simulink model "PSK8"  (R2017a)
settings: Solver=VariableStepAuto  StartTime=0.0  StopTime=9600*Tb  RelTol=1e-3
values from neighbouring files (symbols this model uses):
  Tb = 5e-8    (= 5e-08)    [cuatrobits.m]    (also in dosbits.m; seisbits.m; tresbits.m)
libraries: commfilt2 x4, commdigbbndpm3 x2, dspsigops x2, simulink x1
settings Model: Creator=se.alfonso  LastModifiedBy=af.diaz16

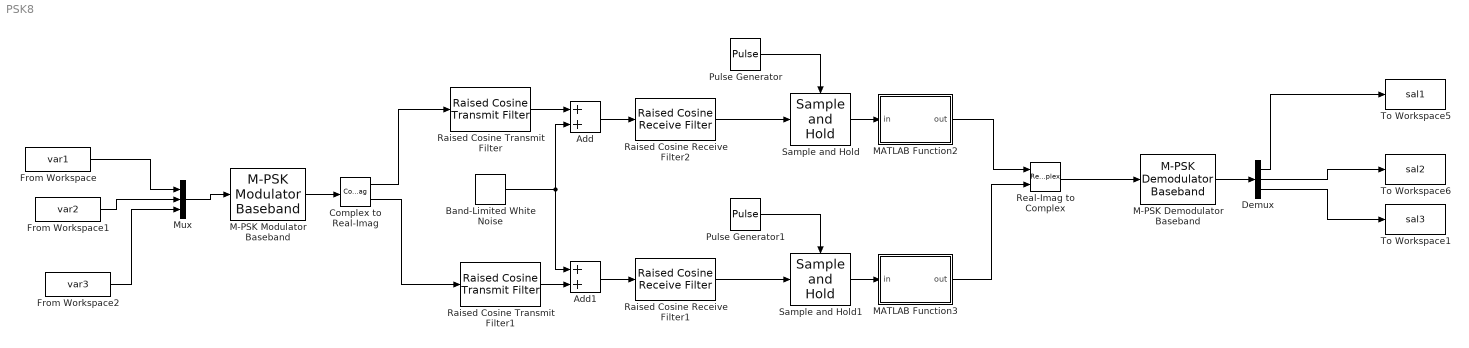
== system PSK8 ==
  Add : Sum
  Add1 : Sum
  Band-Limited White Noise : simulink/Sources/Band-Limited White Noise  Cov=No  Ts=Tb  seed=[23341]
  Complex to Real-Imag : ComplexToRealImag
  Demux : Demux  Outputs=3
  From Workspace : FromWorkspace  VariableName=var1  SampleTime=Tb
  From Workspace1 : FromWorkspace  VariableName=var2  SampleTime=Tb
  From Workspace2 : FromWorkspace  VariableName=var3  SampleTime=Tb
  M-PSK Demodulator Baseband : commdigbbndpm3/M-PSK Demodulator Baseband  M=8  OutType=Bit  DecType=Hard decision  VarSource=Dialog  Variance=1  Dec=Gray  Mapping=[0:7]  Ph=pi/8  outDtype1=Inherit via internal rule  outDtype2=Inherit via internal rule  derotateFactorWordLen=16  derotateFactorDataTypeStr=Inherit: Same word length as input  derotateFactorLastDataTypeStr=Inherit: Same word length as input
      settings: SourceProductName=Communications System Toolbox
  M-PSK Modulator Baseband : commdigbbndpm3/M-PSK Modulator Baseband  M=8  InType=Bit  Enc=Gray  Mapping=[0:7]  Ph=pi/8  outDtype=double  outWordLen=16  outUDDataType=sfix(16)  outFracLenMode=Best precision  outFracLen=15  outDataTypeStr=double  outLastDataTypeStr=double
      settings: SourceProductName=Communications System Toolbox
  MATLAB Function2 : MATLAB Function  TreatAsAtomicUnit=on
  MATLAB Function3 : MATLAB Function  TreatAsAtomicUnit=on
  Mux : Mux  Inputs=3
  Pulse Generator : DiscretePulseGenerator  PulseType=Time based  Period=3*Tb  PulseWidth=50
  Pulse Generator1 : DiscretePulseGenerator  PulseType=Time based  Period=3*Tb  PulseWidth=50
  Raised Cosine Receive Filter1 : commfilt2/Raised Cosine Receive Filter  filtType=Square root  R=0.25  filtSpan=2  N=5  downFactor=1  downOffset=0  filterGain=1  RateOptions=Allow multirate processing  framing=Allow multirate processing  checkCoeff=off  variableName=rcRxFilt1  currentFiltSpan=2  D=(2)/2  inputOffset=0  sampMode=Mute  saveAsFlag=1  rateMode=Downsampling  checkGain=Normalized  launchFVT=on  roundingMode=Floor  overflowMode=off  coeffDataTypeStr=Inherit: Same word length as input  coeffMin=[]  coeffMax=[]  coeffLastDataTypeStr=Inherit: Same word length as input  accumDataTypeStr=Inherit: Same as product output  accumLastDataTypeStr=Inherit: Same as product output  outputDataTypeStr=Inherit: Same as accumulator  outputMin=[]  outputMax=[]  outputLastDataTypeStr=Inherit: Same as accumulator
  Raised Cosine Receive Filter2 : commfilt2/Raised Cosine Receive Filter  filtType=Square root  R=0.25  filtSpan=2  N=5  downFactor=1  downOffset=0  filterGain=1  RateOptions=Allow multirate processing  framing=Allow multirate processing  checkCoeff=off  variableName=rcRxFilt2  currentFiltSpan=2  D=(2)/2  inputOffset=0  sampMode=Mute  saveAsFlag=1  rateMode=Downsampling  checkGain=Normalized  launchFVT=on  roundingMode=Floor  overflowMode=off  coeffDataTypeStr=Inherit: Same word length as input  coeffMin=[]  coeffMax=[]  coeffLastDataTypeStr=Inherit: Same word length as input  accumDataTypeStr=Inherit: Same as product output  accumLastDataTypeStr=Inherit: Same as product output  outputDataTypeStr=Inherit: Same as accumulator  outputMin=[]  outputMax=[]  outputLastDataTypeStr=Inherit: Same as accumulator
  Raised Cosine Transmit Filter : commfilt2/Raised Cosine Transmit Filter  filtType=Square root  R=0.25  filtSpan=2  N=6  filterGain=1  RateOptions=Allow multirate processing  framing=Allow multirate processing  checkCoeff=off  variableName=rcTxFilt  checkGain=Normalized  sampMode=Mute  saveAsFlag=1  currentFiltSpan=2  D=(2)/2  launchFVT=on  roundingMode=Floor  overflowMode=off  coeffDataTypeStr=Inherit: Same word length as input  coeffMin=[]  coeffMax=[]  coeffLastDataTypeStr=Inherit: Same word length as input  outputDataTypeStr=Inherit: Same as accumulator  outputMin=[]  outputMax=[]  outputLastDataTypeStr=Inherit: Same as accumulator
  Raised Cosine Transmit Filter1 : commfilt2/Raised Cosine Transmit Filter  filtType=Square root  R=0.25  filtSpan=2  N=6  filterGain=1  RateOptions=Allow multirate processing  framing=Allow multirate processing  checkCoeff=off  variableName=rcTxFilt1  checkGain=Normalized  sampMode=Mute  saveAsFlag=1  currentFiltSpan=2  D=(2)/2  launchFVT=on  roundingMode=Floor  overflowMode=off  coeffDataTypeStr=Inherit: Same word length as input  coeffMin=[]  coeffMax=[]  coeffLastDataTypeStr=Inherit: Same word length as input  outputDataTypeStr=Inherit: Same as accumulator  outputMin=[]  outputMax=[]  outputLastDataTypeStr=Inherit: Same as accumulator
  Real-Imag to Complex : RealImagToComplex
  Sample and Hold : dspsigops/Sample and Hold  trig=Rising edge  initCond=0  latchinput=off
  Sample and Hold1 : dspsigops/Sample and Hold  trig=Rising edge  initCond=0  latchinput=off
  To Workspace1 : ToWorkspace  VariableName=sal3  SampleTime=Tb
      settings: Save2DSignal=2-D array (concatenate along first dimension)
  To Workspace5 : ToWorkspace  VariableName=sal1  SampleTime=Tb
      settings: Save2DSignal=2-D array (concatenate along first dimension)
  To Workspace6 : ToWorkspace  VariableName=sal2  SampleTime=Tb
      settings: Save2DSignal=2-D array (concatenate along first dimension)
  wires:
  From Workspace1/1 -> Mux/2
  Complex to Real-Imag/1 -> Raised Cosine Transmit Filter/1
  Raised Cosine Transmit Filter/1 -> Add/1
  Band-Limited White Noise/1 -> Add/2, Add1/1
  Add/1 -> Raised Cosine Receive Filter2/1
  Demux/1 -> To Workspace5/1
  Complex to Real-Imag/2 -> Raised Cosine Transmit Filter1/1
  M-PSK Demodulator Baseband/1 -> Demux/1
  Demux/2 -> To Workspace6/1
  Pulse Generator1/1 -> Sample and Hold1/Trigger
  Raised Cosine Receive Filter2/1 -> Sample and Hold/1
  Pulse Generator/1 -> Sample and Hold/Trigger
  Add1/1 -> Raised Cosine Receive Filter1/1
  From Workspace/1 -> Mux/1
  Raised Cosine Transmit Filter1/1 -> Add1/2
  Mux/1 -> M-PSK Modulator Baseband/1
  M-PSK Modulator Baseband/1 -> Complex to Real-Imag/1
  Raised Cosine Receive Filter1/1 -> Sample and Hold1/1
  From Workspace2/1 -> Mux/3
  Demux/3 -> To Workspace1/1
  Real-Imag to Complex/1 -> M-PSK Demodulator Baseband/1
  Sample and Hold1/1 -> MATLAB Function3/1(in)
  Sample and Hold/1 -> MATLAB Function2/1(in)
  MATLAB Function2/1(out) -> Real-Imag to Complex/1
  MATLAB Function3/1(out) -> Real-Imag to Complex/2

== matlab function PSK8/MATLAB Function2 ==
  data: in input; out output
function out   = DecisionReal(in)

out=zeros(size(in),'like',in);

niv=1:4;
niv(1)=-real(1*exp(j*pi/8));
niv(2)=-real(1*exp(j*3*pi/8));
niv(3)=real(1*exp(j*3*pi/8));
niv(4)=real(1*exp(j*pi/8));

if in < 0
    if in < -0.6533
    out=niv(1);
    end
    if in >= -0.6533
    out=niv(2);
    end
end
if in >= 0
    if in < 0.6533 
    out=niv(3);
    end
    if in >= 0.6533
    out=niv(4);
    end
end    
end

== matlab function PSK8/MATLAB Function3 ==
  data: in input; out output
function out = DecisionIm(in)

out=zeros(size(in),'like',in);

niv=1:4;
niv(1)=-real(1*exp(j*pi/8));
niv(2)=-real(1*exp(j*3*pi/8));
niv(3)=real(1*exp(j*3*pi/8));
niv(4)=real(1*exp(j*pi/8));

if in < 0
    if in < -0.6533
    out=niv(1);
    end
    if in >= -0.6533
    out=niv(2);
    end
end
if in >= 0
    if in < 0.6533 
    out=niv(3);
    end
    if in >= 0.6533
    out=niv(4);
    end
end    
end
